simulink model "PV_system0000"  (R2016a)
settings: Solver=VariableStepAuto  StartTime=0.0  StopTime=0.6001  RelTol=1e-3
libraries: powerlib x6, re_lib x1, simulink x1
settings Model: Creator=Rafi  LastModifiedBy=Emdadul Haq

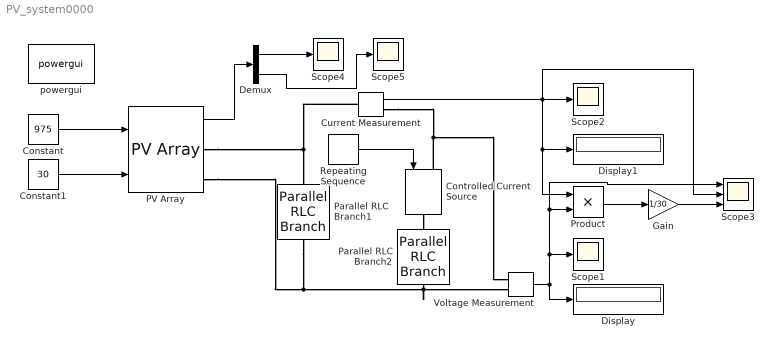
== system PV_system0000 ==
  Constant : Constant  Value=975
  Constant1 : Constant  Value=30
  Controlled Current Source : powerlib/Electrical Sources/Controlled Current Source  Initialize=on  Source_Type=DC  Amplitude=0  Phase=0  Frequency=0  Measurements=Current
  Current Measurement : powerlib/Measurements/Current Measurement  PhasorSimulation=off  OutputType=Complex  PSBequivalent=0
  Demux : Demux  Outputs=2
  Display : Display
  Display1 : Display
  Gain : Gain  Gain=1/30
  PV Array : re_lib/Solar/PV Array  Npar=10  Nser=1  PlotType=array @ 1000 W/m2 & specified temperatures  S_vec="[ 1000  500  100 ]"  Temp_C_vec="[ 45 25  ]"  ModuleName=1Soltech 1STH-215-P  PlotWhenSelected=off  Pm=213.15  Ncell=60  Voc=36.3  Isc=7.84  Vm=29  Im=7.35  beta_Voc_pc=-0.36099  alpha_Isc_pc=0.102  beta_Voc=-0.13104  alpha_Isc=0.007997  IL=7.8649  I0=2.9259e-10  nI=0.98117  Rsh=313.3991  Rs=0.39383  BAL=off  Tc=1e-6  Tfilter=5e-5
  Parallel RLC Branch1 : powerlib/Elements/Parallel RLC Branch  LConnTagsString=a  RConnTagsString=__new0  BranchType=C  Resistance=1  Inductance=1e-3  SetiL0=off  InitialCurrent=0  Capacitance=1000e-6  Setx0=off  InitialVoltage=0  Measurements=None
  Parallel RLC Branch2 : powerlib/Elements/Parallel RLC Branch  LConnTagsString=a  RConnTagsString=__new0  BranchType=R  Resistance=5  Inductance=1e-3  SetiL0=off  InitialCurrent=0  Capacitance=470e-6  Setx0=off  InitialVoltage=0  Measurements=None
  Product : Product
  Repeating Sequence : simulink/Sources/Repeating Sequence  rep_seq_t=[0 0.6]  rep_seq_y=[0 79]
  Scope{1..2,4..5} (4 alike) : Scope
  Scope3 : Scope  NumInputPorts=3
  Voltage Measurement : powerlib/Measurements/Voltage Measurement  PhasorSimulation=off  OutputType=Complex  PSBequivalent=0
  powergui : powerlib/powergui  Priority=1  SimulationMode=Continuous  SolverType=Tustin/Backward Euler (TBE)  SampleTime=50e-6  frequency=60  SPID=off  DisableSnubberDevices=off  DisableRonSwitches=off  DisableVfSwitches=off  SwTol=0  DisplayEquations=off  Interpol=off  ExternalGateDelay=off  methode=off  Ts=10  FunctionMessages=off  echomessages=off  HookPort=off  EnableUseOfTLC=off  x0status=blocks  frequencyindice=0  Pbase=100e6  ErrMax=1e-4  Iterations=50  UnitsV=kV  UnitsW=MW  buscounter=0  RestoreLinks=warning  ResistiveCurrentMeasurement=off  Frange=[0:2:500]  Ylog=off  Xlog=on  ShowGrid=off  save=off  variable=ZData  structure=0  ZoomFFT=off  StartTime=0.0  cycles=1  DisplayStyle=1  fundamental=60  FreqAxis=off  MaxFrequency=1000  frequencyindicesteady=1  RmsSteady=1  display=off
  wires:
  Constant/1 -> PV Array/1
  Constant1/1 -> PV Array/2
  Voltage Measurement/1 -> Scope3/1, Product/2, Scope1/1, Display/1
  Repeating Sequence/1 -> Controlled Current Source/1
  PV Array/1 -> Demux/1
  Demux/1 -> Scope4/1
  Demux/2 -> Scope5/1
  Product/1 -> Gain/1
  Current Measurement/1 -> Scope2/1, Scope3/2, Display1/1, Product/1
  Gain/1 -> Scope3/3
  connections:
  PV Array/RConn2 -- Parallel RLC Branch2/RConn1 -- Voltage Measurement/LConn2 -- Parallel RLC Branch1/RConn1
  PV Array/RConn1 -- Current Measurement/LConn1 -- Parallel RLC Branch1/LConn1
  Current Measurement/RConn1 -- Voltage Measurement/LConn1 -- Controlled Current Source/LConn1
  Controlled Current Source/RConn1 -- Parallel RLC Branch2/LConn1
